simulink model "FeedbackControl"  (R2023a)
settings: Solver=VariableStepAuto  StartTime=0.0  StopTime=10.0  RelTol=1e-3
settings Model: Creator=aan18022  LastModifiedBy=aan18022

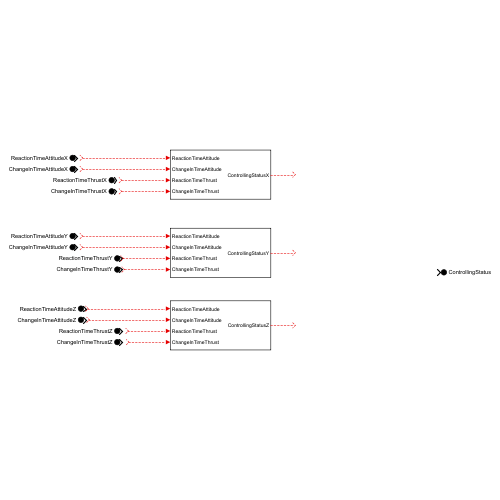
[thumbnail: Simulink's stored preview of the top-level diagram]
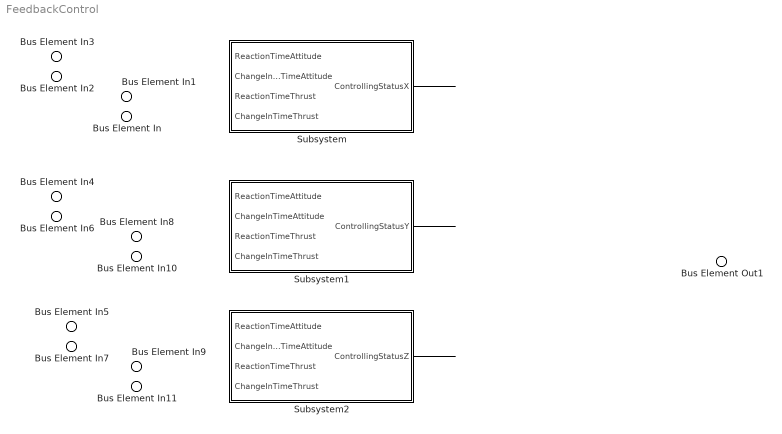
== system FeedbackControl ==
  Bus Element In2 : Inport  PortName=ChangeInTimeAttitudeX
  Bus Element In1 : Inport  Port=2  PortName=ReactionTimeThrustX
  Bus Element In : Inport  Port=3  PortName=ChangeInTimeThrustX
  Bus Element In3 : Inport  Port=4  PortName=ReactionTimeAttitudeX
  Bus Element In4 : Inport  Port=5  PortName=ReactionTimeAttitudeY
  Bus Element In5 : Inport  Port=6  PortName=ReactionTimeAttitudeZ
  Bus Element In6 : Inport  Port=7  PortName=ChangeInTimeAttitudeY
  Bus Element In7 : Inport  Port=8  PortName=ChangeInTimeAttitudeZ
  Bus Element In8 : Inport  Port=9  PortName=ReactionTimeThrustY
  Bus Element In9 : Inport  Port=10  PortName=ReactionTimeThrustZ
  Bus Element In10 : Inport  Port=11  PortName=ChangeInTimeThrustY
  Bus Element In11 : Inport  Port=12  PortName=ChangeInTimeThrustZ
  Subsystem : Subsystem
  Subsystem1 : Subsystem
  Subsystem2 : Subsystem
  Bus Element Out1 : Outport  PortName=ControllingStatus
  wires:
  ? -> Subsystem/3(ReactionTimeThrust)
  ? -> Subsystem/1(ReactionTimeAttitude)
  Subsystem/1(ControllingStatusX) -> ?
  ? -> Subsystem/4(ChangeInTimeThrust)
  ? -> Subsystem/2(ChangeInTimeAttitude)
  ? -> Subsystem1/2(ChangeInTimeAttitude)
  ? -> Subsystem1/3(ReactionTimeThrust)
  ? -> Subsystem1/1(ReactionTimeAttitude)
  ? -> Subsystem1/4(ChangeInTimeThrust)
  Subsystem1/1(ControllingStatusY) -> ?
  ? -> Subsystem2/2(ChangeInTimeAttitude)
  ? -> Subsystem2/1(ReactionTimeAttitude)
  Subsystem2/1(ControllingStatusZ) -> ?
  ? -> Subsystem2/3(ReactionTimeThrust)
  ? -> Subsystem2/4(ChangeInTimeThrust)

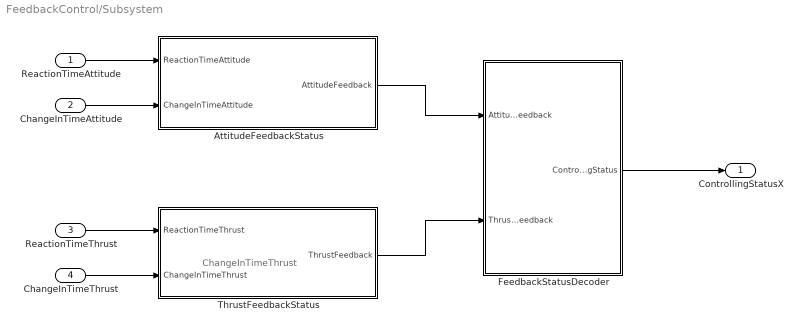
== system FeedbackControl/Subsystem ==
  note: ChangeInTimeThrust
  ReactionTimeAttitude : Inport
  ChangeInTimeAttitude : Inport  Port=2
  ReactionTimeThrust : Inport  Port=3
  ChangeInTimeThrust : Inport  Port=4
  AttitudeFeedbackStatus : Subsystem
  FeedbackStatusDecoder : Subsystem
  ThrustFeedbackStatus : Subsystem
  ControllingStatusX : Outport
  wires:
  ReactionTimeThrust/1 -> ThrustFeedbackStatus/1(ReactionTimeThrust)
  ChangeInTimeThrust/1 -> ThrustFeedbackStatus/2(ChangeInTimeThrust)
  ChangeInTimeAttitude/1 -> AttitudeFeedbackStatus/2(ChangeInTimeAttitude)
  ReactionTimeAttitude/1 -> AttitudeFeedbackStatus/1(ReactionTimeAttitude)
  ThrustFeedbackStatus/1(ThrustFeedback) -> FeedbackStatusDecoder/2(ThrustFeedback)
  AttitudeFeedbackStatus/1(AttitudeFeedback) -> FeedbackStatusDecoder/1(AttitudeFeedback)
  FeedbackStatusDecoder/1(ControllingStatus) -> ControllingStatusX/1

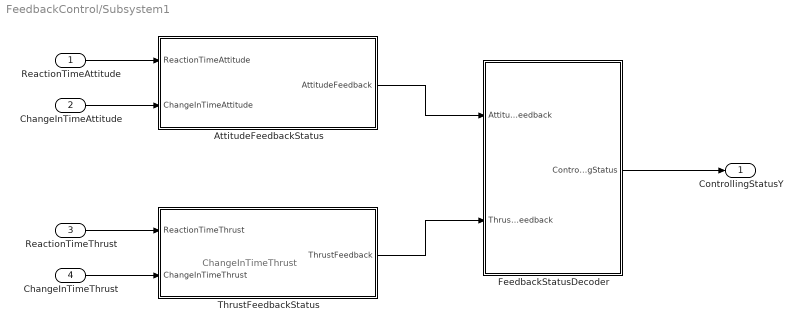
== system FeedbackControl/Subsystem1 ==
  note: ChangeInTimeThrust
  ReactionTimeAttitude : Inport
  ChangeInTimeAttitude : Inport  Port=2
  ReactionTimeThrust : Inport  Port=3
  ChangeInTimeThrust : Inport  Port=4
  AttitudeFeedbackStatus : Subsystem
  FeedbackStatusDecoder : Subsystem
  ThrustFeedbackStatus : Subsystem
  ControllingStatusY : Outport
  wires:
  ReactionTimeThrust/1 -> ThrustFeedbackStatus/1(ReactionTimeThrust)
  ChangeInTimeThrust/1 -> ThrustFeedbackStatus/2(ChangeInTimeThrust)
  ChangeInTimeAttitude/1 -> AttitudeFeedbackStatus/2(ChangeInTimeAttitude)
  ReactionTimeAttitude/1 -> AttitudeFeedbackStatus/1(ReactionTimeAttitude)
  ThrustFeedbackStatus/1(ThrustFeedback) -> FeedbackStatusDecoder/2(ThrustFeedback)
  AttitudeFeedbackStatus/1(AttitudeFeedback) -> FeedbackStatusDecoder/1(AttitudeFeedback)
  FeedbackStatusDecoder/1(ControllingStatus) -> ControllingStatusY/1

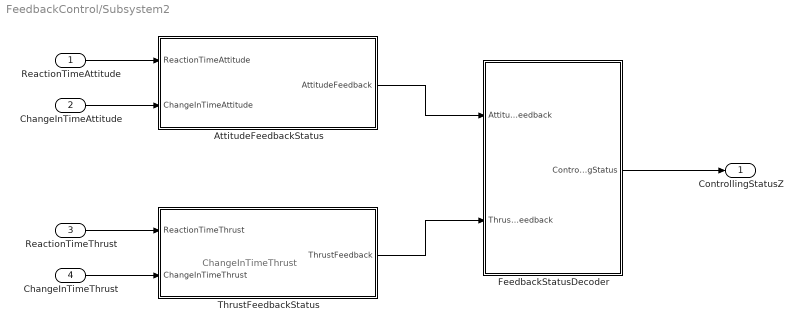
== system FeedbackControl/Subsystem2 ==
  note: ChangeInTimeThrust
  ReactionTimeAttitude : Inport
  ChangeInTimeAttitude : Inport  Port=2
  ReactionTimeThrust : Inport  Port=3
  ChangeInTimeThrust : Inport  Port=4
  AttitudeFeedbackStatus : Subsystem
  FeedbackStatusDecoder : Subsystem
  ThrustFeedbackStatus : Subsystem
  ControllingStatusZ : Outport
  wires:
  ReactionTimeThrust/1 -> ThrustFeedbackStatus/1(ReactionTimeThrust)
  ChangeInTimeThrust/1 -> ThrustFeedbackStatus/2(ChangeInTimeThrust)
  ChangeInTimeAttitude/1 -> AttitudeFeedbackStatus/2(ChangeInTimeAttitude)
  ReactionTimeAttitude/1 -> AttitudeFeedbackStatus/1(ReactionTimeAttitude)
  ThrustFeedbackStatus/1(ThrustFeedback) -> FeedbackStatusDecoder/2(ThrustFeedback)
  AttitudeFeedbackStatus/1(AttitudeFeedback) -> FeedbackStatusDecoder/1(AttitudeFeedback)
  FeedbackStatusDecoder/1(ControllingStatus) -> ControllingStatusZ/1

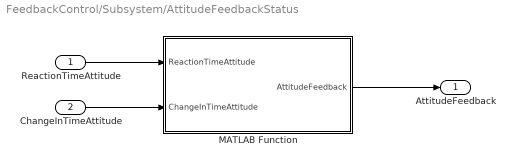
== system FeedbackControl/Subsystem/AttitudeFeedbackStatus ==
  ReactionTimeAttitude : Inport
  ChangeInTimeAttitude : Inport  Port=2
  MATLAB Function : MATLAB Function  TreatAsAtomicUnit=on
  AttitudeFeedback : Outport
  wires:
  ChangeInTimeAttitude/1 -> MATLAB Function/2(ChangeInTimeAttitude)
  ReactionTimeAttitude/1 -> MATLAB Function/1(ReactionTimeAttitude)
  MATLAB Function/1(AttitudeFeedback) -> AttitudeFeedback/1

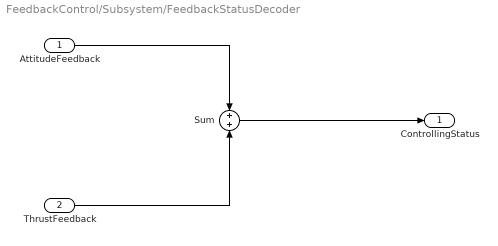
== system FeedbackControl/Subsystem/FeedbackStatusDecoder ==
  AttitudeFeedback : Inport
  ThrustFeedback : Inport  Port=2
  Sum : Sum
  ControllingStatus : Outport
  wires:
  ThrustFeedback/1 -> Sum/2
  AttitudeFeedback/1 -> Sum/1
  Sum/1 -> ControllingStatus/1

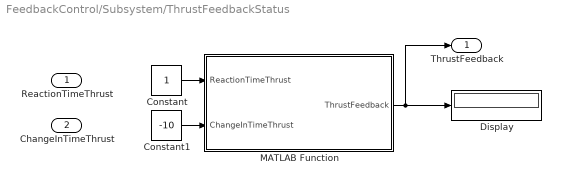
== system FeedbackControl/Subsystem/ThrustFeedbackStatus ==
  ReactionTimeThrust : Inport
  ChangeInTimeThrust : Inport  Port=2
  Constant : Constant
  Constant1 : Constant  Value=-10
  Display : Display
  MATLAB Function : MATLAB Function  TreatAsAtomicUnit=on
  ThrustFeedback : Outport
  wires:
  MATLAB Function/1(ThrustFeedback) -> ThrustFeedback/1, Display/1
  Constant/1 -> MATLAB Function/1(ReactionTimeThrust)
  Constant1/1 -> MATLAB Function/2(ChangeInTimeThrust)

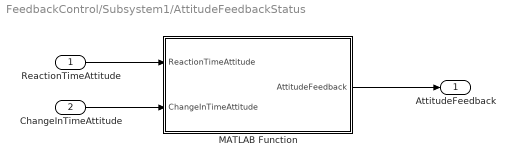
== system FeedbackControl/Subsystem1/AttitudeFeedbackStatus ==
  ReactionTimeAttitude : Inport
  ChangeInTimeAttitude : Inport  Port=2
  MATLAB Function : MATLAB Function  TreatAsAtomicUnit=on
  AttitudeFeedback : Outport
  wires:
  ChangeInTimeAttitude/1 -> MATLAB Function/2(ChangeInTimeAttitude)
  ReactionTimeAttitude/1 -> MATLAB Function/1(ReactionTimeAttitude)
  MATLAB Function/1(AttitudeFeedback) -> AttitudeFeedback/1

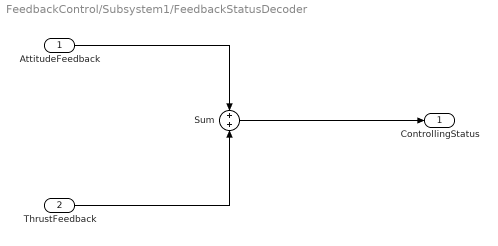
== system FeedbackControl/Subsystem1/FeedbackStatusDecoder ==
  AttitudeFeedback : Inport
  ThrustFeedback : Inport  Port=2
  Sum : Sum
  ControllingStatus : Outport
  wires:
  ThrustFeedback/1 -> Sum/2
  AttitudeFeedback/1 -> Sum/1
  Sum/1 -> ControllingStatus/1

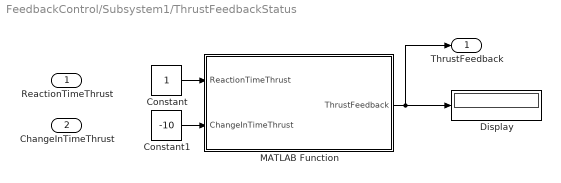
== system FeedbackControl/Subsystem1/ThrustFeedbackStatus ==
  ReactionTimeThrust : Inport
  ChangeInTimeThrust : Inport  Port=2
  Constant : Constant
  Constant1 : Constant  Value=-10
  Display : Display
  MATLAB Function : MATLAB Function  TreatAsAtomicUnit=on
  ThrustFeedback : Outport
  wires:
  MATLAB Function/1(ThrustFeedback) -> ThrustFeedback/1, Display/1
  Constant/1 -> MATLAB Function/1(ReactionTimeThrust)
  Constant1/1 -> MATLAB Function/2(ChangeInTimeThrust)

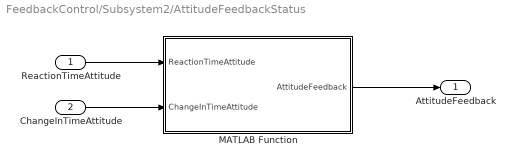
== system FeedbackControl/Subsystem2/AttitudeFeedbackStatus ==
  ReactionTimeAttitude : Inport
  ChangeInTimeAttitude : Inport  Port=2
  MATLAB Function : MATLAB Function  TreatAsAtomicUnit=on
  AttitudeFeedback : Outport
  wires:
  ChangeInTimeAttitude/1 -> MATLAB Function/2(ChangeInTimeAttitude)
  ReactionTimeAttitude/1 -> MATLAB Function/1(ReactionTimeAttitude)
  MATLAB Function/1(AttitudeFeedback) -> AttitudeFeedback/1

== system FeedbackControl/Subsystem2/FeedbackStatusDecoder ==
  AttitudeFeedback : Inport
  ThrustFeedback : Inport  Port=2
  Sum : Sum
  ControllingStatus : Outport
  wires:
  ThrustFeedback/1 -> Sum/2
  AttitudeFeedback/1 -> Sum/1
  Sum/1 -> ControllingStatus/1

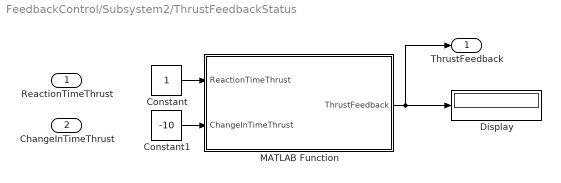
== system FeedbackControl/Subsystem2/ThrustFeedbackStatus ==
  ReactionTimeThrust : Inport
  ChangeInTimeThrust : Inport  Port=2
  Constant : Constant
  Constant1 : Constant  Value=-10
  Display : Display
  MATLAB Function : MATLAB Function  TreatAsAtomicUnit=on
  ThrustFeedback : Outport
  wires:
  MATLAB Function/1(ThrustFeedback) -> ThrustFeedback/1, Display/1
  Constant/1 -> MATLAB Function/1(ReactionTimeThrust)
  Constant1/1 -> MATLAB Function/2(ChangeInTimeThrust)

== matlab function FeedbackControl/Subsystem/ThrustFeedbackStatus/MATLAB Function ==
  data: ReactionTimeThrust input; ChangeInTimeThrust input; ThrustFeedback output
function ThrustFeedback = fcn(ReactionTimeThrust, ChangeInTimeThrust)

if ChangeInTimeThrust == -10
    ThrustFeedback = 1000 + ReactionTimeThrust;
else
    ThrustFeedback = 0;
end

== matlab function FeedbackControl/Subsystem1/AttitudeFeedbackStatus/MATLAB Function ==
  data: ReactionTimeAttitude input; ChangeInTimeAttitude input; AttitudeFeedback output
function AttitudeFeedback = fcn(ReactionTimeAttitude, ChangeInTimeAttitude)

if ChangeInTimeAttitude == -10
    AttitudeFeedback = 2000 + ReactionTimeAttitude;
else
    AttitudeFeedback = 0;
end

== matlab function FeedbackControl/Subsystem1/ThrustFeedbackStatus/MATLAB Function ==
  data: ReactionTimeThrust input; ChangeInTimeThrust input; ThrustFeedback output
function ThrustFeedback = fcn(ReactionTimeThrust, ChangeInTimeThrust)

if ChangeInTimeThrust == -10
    ThrustFeedback = 1000 + ReactionTimeThrust;
else
    ThrustFeedback = 0;
end

== matlab function FeedbackControl/Subsystem2/AttitudeFeedbackStatus/MATLAB Function ==
  data: ReactionTimeAttitude input; ChangeInTimeAttitude input; AttitudeFeedback output
function AttitudeFeedback = fcn(ReactionTimeAttitude, ChangeInTimeAttitude)

if ChangeInTimeAttitude == -10
    AttitudeFeedback = 2000 + ReactionTimeAttitude;
else
    AttitudeFeedback = 0;
end

== matlab function FeedbackControl/Subsystem2/ThrustFeedbackStatus/MATLAB Function ==
  data: ReactionTimeThrust input; ChangeInTimeThrust input; ThrustFeedback output
function ThrustFeedback = fcn(ReactionTimeThrust, ChangeInTimeThrust)

if ChangeInTimeThrust == -10
    ThrustFeedback = 1000 + ReactionTimeThrust;
else
    ThrustFeedback = 0;
end

== matlab function FeedbackControl/Subsystem/AttitudeFeedbackStatus/MATLAB Function ==
  data: ReactionTimeAttitude input; ChangeInTimeAttitude input; AttitudeFeedback output
function AttitudeFeedback = fcn(ReactionTimeAttitude, ChangeInTimeAttitude)

if ChangeInTimeAttitude == -10
    AttitudeFeedback = 2000 + ReactionTimeAttitude;
else
    AttitudeFeedback = 0;
end
